simulink model "Controller"  (R2020b)
settings: Solver=FixedStepDiscrete  StartTime=0.0  StopTime=10.0  FixedStep=controllerSampleTime  RelTol=1e-3
values from neighbouring files (symbols this model uses):
  eetaRoad = 5.0    [AOTDataDictionary.sldd]
  egoAccMax = 5.0    [AOTDataDictionary.sldd]
  egoAccMin = -10.0    [AOTDataDictionary.sldd]
  egoSteerAngMax = 0.52359877559829882    [AOTDataDictionary.sldd]
  egoSteerAngMin = -0.52359877559829882    [AOTDataDictionary.sldd]
  egoVehLength = 4.948    [AOTDataDictionary.sldd]
  egoVehWidth = 2.009    [AOTDataDictionary.sldd]
  inflation_factor = 1.0    [AOTDataDictionary.sldd]
  L = 3.705    [AOTDataDictionary.sldd]
  l_F = 1.2525    [AOTDataDictionary.sldd]
  npcVehLength = 4.848    [AOTDataDictionary.sldd]
  npcVehWidth = 1.842    [AOTDataDictionary.sldd]
  obstcl_ellip_order = 6.0    [AOTDataDictionary.sldd]
  ReachableSetCurveResolution = 0.1    [AOTDataDictionary.sldd]
  RiskMaxValue = 100.0    [AOTDataDictionary.sldd]
  RiskValueThreshold = 15.0    [AOTDataDictionary.sldd]
  SenseResolution = 0.1    [AOTDataDictionary.sldd]
  v_des = 8.0    [AOTDataDictionary.sldd]
  XSenseRange = 20.0    [AOTDataDictionary.sldd]
  XSenseRangeArrSize = 401.0    [AOTDataDictionary.sldd]
  YSenseRange = 20.0    [AOTDataDictionary.sldd]
  YSenseRangeArrSize = 401.0    [AOTDataDictionary.sldd]
undefined symbols (not defined in the file or in its folder): VEH
libraries: mpclib x1, autolibshared x1, vehdynlibdriver x1
settings Model: DataDictionary=AOTDataDictionary.sldd  Creator=jiyoj  LastModifiedBy=jiyoj
settings DataIOCC: SaveOutput=off  SignalLogging=off  DSMLogging=off  SaveTime=off  ReturnWorkspaceOutputs=off

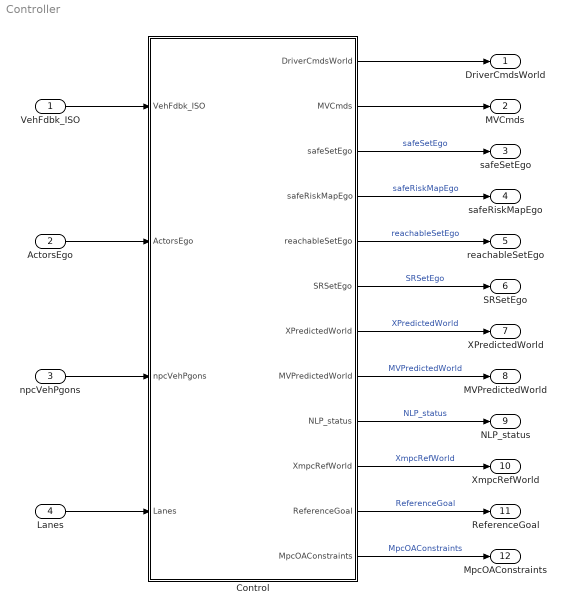
== system Controller ==
  VehFdbk_ISO : Inport  OutDataTypeStr=Bus: Veh_Fdbk  BusOutputAsStruct=on
  ActorsEgo : Inport  Port=2  OutDataTypeStr=Bus: BusActors  PortDimensions=[1 1]  BusOutputAsStruct=on
  npcVehPgons : Inport  Port=3  OutDataTypeStr=Bus: VehPgons  BusOutputAsStruct=on
  Lanes : Inport  Port=4  OutDataTypeStr=Bus: BusLaneBoundaries  PortDimensions=[1 1]  BusOutputAsStruct=on
  Control : Subsystem
  DriverCmdsWorld : Outport  OutDataTypeStr=Bus: DriverCmd  BusOutputAsStruct=on
  MVCmds : Outport  Port=2
  safeSetEgo : Outport  Port=3
  safeRiskMapEgo : Outport  Port=4
  reachableSetEgo : Outport  Port=5
  SRSetEgo : Outport  Port=6
  XPredictedWorld : Outport  Port=7
  MVPredictedWorld : Outport  Port=8
  NLP_status : Outport  Port=9
  XmpcRefWorld : Outport  Port=10
  ReferenceGoal : Outport  Port=11  OutDataTypeStr=Bus: Position2D  BusOutputAsStruct=on
  MpcOAConstraints : Outport  Port=12
  wires:
  VehFdbk_ISO/1 -> Control/1(VehFdbk_ISO)
  ActorsEgo/1 -> Control/2(ActorsEgo)
  Lanes/1 -> Control/4(Lanes)
  Control/1(DriverCmdsWorld) -> DriverCmdsWorld/1
  Control/3(safeSetEgo) -> safeSetEgo/1  "safeSetEgo"
  Control/4(safeRiskMapEgo) -> safeRiskMapEgo/1  "safeRiskMapEgo"
  npcVehPgons/1 -> Control/3(npcVehPgons)
  Control/5(reachableSetEgo) -> reachableSetEgo/1  "reachableSetEgo"
  Control/6(SRSetEgo) -> SRSetEgo/1  "SRSetEgo"
  Control/7(XPredictedWorld) -> XPredictedWorld/1  "XPredictedWorld"
  Control/8(MVPredictedWorld) -> MVPredictedWorld/1  "MVPredictedWorld"
  Control/9(NLP_status) -> NLP_status/1  "NLP_status"
  Control/10(XmpcRefWorld) -> XmpcRefWorld/1  "XmpcRefWorld"
  Control/11(ReferenceGoal) -> ReferenceGoal/1  "ReferenceGoal"
  Control/12(MpcOAConstraints) -> MpcOAConstraints/1  "MpcOAConstraints"
  Control/2(MVCmds) -> MVCmds/1

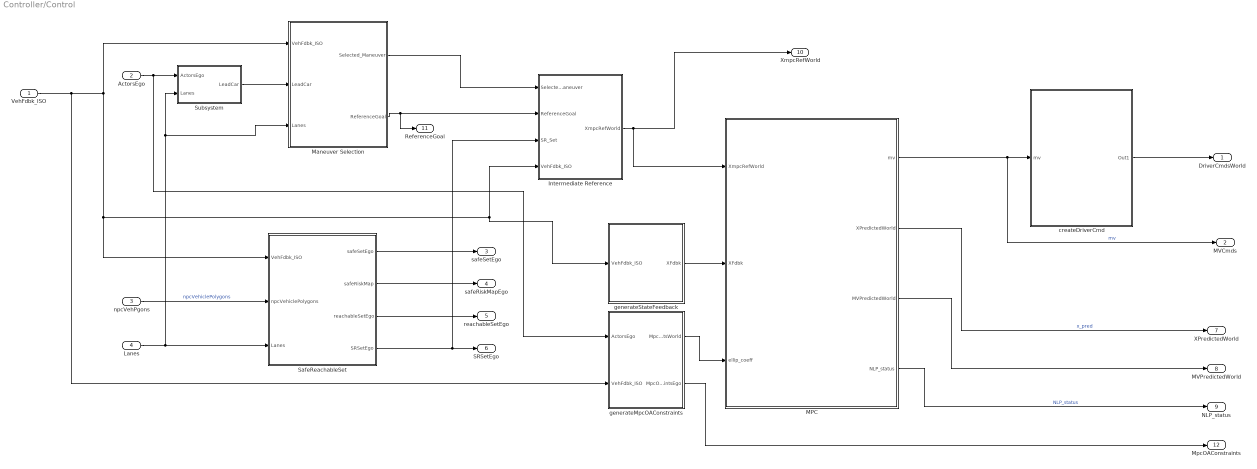
== system Controller/Control ==
  VehFdbk_ISO : Inport
  ActorsEgo : Inport  Port=2
  npcVehPgons : Inport  Port=3
  Lanes : Inport  Port=4
  Intermediate Reference : Subsystem
  MPC : Subsystem
  Maneuver Selection : Subsystem
  SafeReachableSet : Subsystem
  Subsystem : Subsystem
  createDriverCmd : Subsystem
  generateMpcOAConstraints : Subsystem
  generateStateFeedback : Subsystem
  DriverCmdsWorld : Outport
  MVCmds : Outport  Port=2
  safeSetEgo : Outport  Port=3
  safeRiskMapEgo : Outport  Port=4
  reachableSetEgo : Outport  Port=5
  SRSetEgo : Outport  Port=6
  XPredictedWorld : Outport  Port=7
  MVPredictedWorld : Outport  Port=8
  NLP_status : Outport  Port=9
  XmpcRefWorld : Outport  Port=10
  ReferenceGoal : Outport  Port=11
  MpcOAConstraints : Outport  Port=12
  wires:
  ActorsEgo/1 -> generateMpcOAConstraints/1(ActorsEgo), Subsystem/1(ActorsEgo)
  Lanes/1 -> SafeReachableSet/3(Lanes), Maneuver Selection/3(Lanes), Subsystem/2(Lanes)
  generateMpcOAConstraints/1(MpcOAConstraintsWorld) -> MPC/3(ellip_coeff)
  Maneuver Selection/1(Selected_Maneuver) -> Intermediate Reference/1(Selected_Maneuver)
  VehFdbk_ISO/1 -> generateMpcOAConstraints/2(VehFdbk_ISO), SafeReachableSet/1(VehFdbk_ISO), generateStateFeedback/1(VehFdbk_ISO), Intermediate Reference/4(VehFdbk_ISO), Maneuver Selection/1(VehFdbk_ISO)
  npcVehPgons/1 -> SafeReachableSet/2(npcVehiclePolygons)  "npcVehiclePolygons"
  SafeReachableSet/1(safeSetEgo) -> safeSetEgo/1
  SafeReachableSet/2(safeRiskMap) -> safeRiskMapEgo/1
  SafeReachableSet/3(reachableSetEgo) -> reachableSetEgo/1
  SafeReachableSet/4(SRSetEgo) -> SRSetEgo/1, Intermediate Reference/3(SR_Set)
  MPC/1(mv) -> MVCmds/1, createDriverCmd/1(mv)  "mv"
  createDriverCmd/1(Out1) -> DriverCmdsWorld/1
  Subsystem/1(LeadCar) -> Maneuver Selection/2(LeadCar)
  MPC/2(XPredictedWorld) -> XPredictedWorld/1  "x_pred"
  MPC/3(MVPredictedWorld) -> MVPredictedWorld/1
  MPC/4(NLP_status) -> NLP_status/1  "NLP_status"
  Maneuver Selection/2(ReferenceGoal) -> ReferenceGoal/1, Intermediate Reference/2(ReferenceGoal)
  generateMpcOAConstraints/2(MpcOAConstraintsEgo) -> MpcOAConstraints/1
  Intermediate Reference/1(XmpcRefWorld) -> MPC/1(XmpcRefWorld), XmpcRefWorld/1
  generateStateFeedback/1(XFdbk) -> MPC/2(XFdbk)

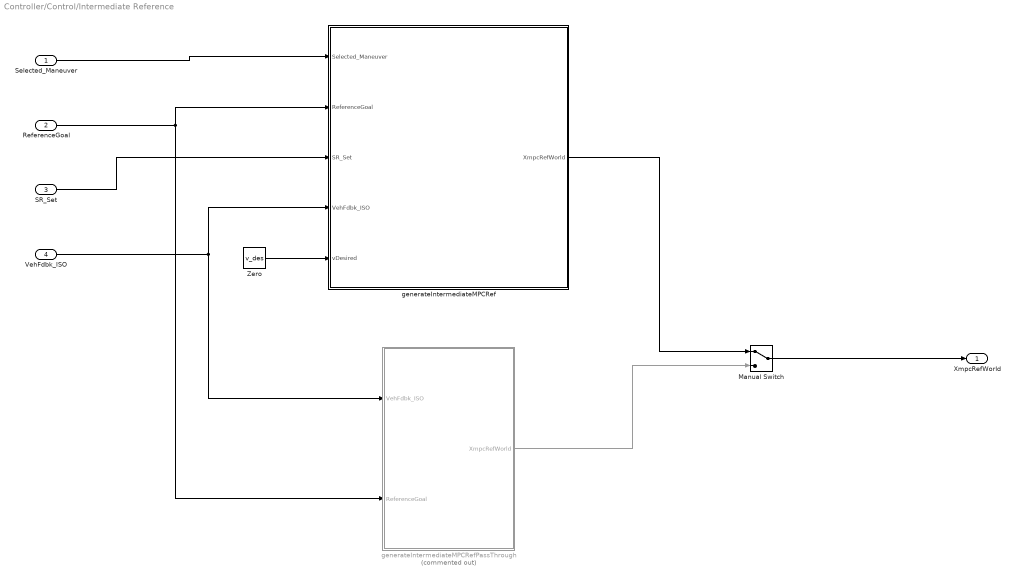
== system Controller/Control/Intermediate Reference ==
  Selected_Maneuver : Inport
  ReferenceGoal : Inport  Port=2
  SR_Set : Inport  Port=3
  VehFdbk_ISO : Inport  Port=4
  Manual Switch : ManualSwitch
  Zero : Constant  Value=v_des  OutDataTypeStr=Inherit: Inherit via back propagation
  generateIntermediateMPCRef : MATLAB Function  TreatAsAtomicUnit=on
  generateIntermediateMPCRefPassThrough : MATLAB Function  Commented=on  TreatAsAtomicUnit=on
  XmpcRefWorld : Outport
  wires:
  Selected_Maneuver/1 -> generateIntermediateMPCRef/1(Selected_Maneuver)
  SR_Set/1 -> generateIntermediateMPCRef/3(SR_Set)
  generateIntermediateMPCRef/1(XmpcRefWorld) -> Manual Switch/1
  ReferenceGoal/1 -> generateIntermediateMPCRefPassThrough/2(ReferenceGoal), generateIntermediateMPCRef/2(ReferenceGoal)
  generateIntermediateMPCRefPassThrough/1(XmpcRefWorld) -> Manual Switch/2
  VehFdbk_ISO/1 -> generateIntermediateMPCRefPassThrough/1(VehFdbk_ISO), generateIntermediateMPCRef/4(VehFdbk_ISO)
  Manual Switch/1 -> XmpcRefWorld/1
  Zero/1 -> generateIntermediateMPCRef/5(vDesired)

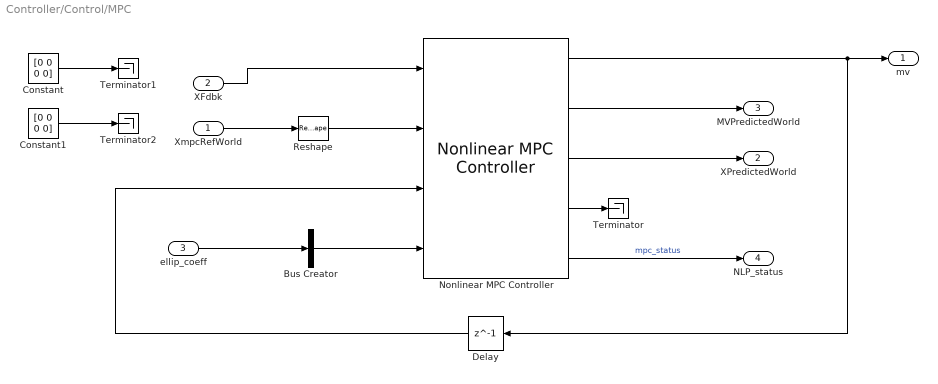
== system Controller/Control/MPC ==
  XmpcRefWorld : Inport
  XFdbk : Inport  Port=2
  ellip_coeff : Inport  Port=3
  Bus Creator : BusCreator  Inputs=1  OutDataTypeStr=Bus: MPCparams  NonVirtualBus=on
      settings: InheritFromInputs=off
  Constant : Constant  Value=[0 0 0 0]
  Constant1 : Constant  Value=[0 0 0 0]
  Delay : Delay  DelayLength=1
  Nonlinear MPC Controller : mpclib/Nonlinear MPC Controller  SCDEnableBlockLinearizationSpecification=on  nlmpcobj=mpc_planner  UseObjectTs=on  TsControl=-1  UseMEX=off  md_enabled=off  mvtarget_enabled=off  param_enabled=on  cost_enabled=off  mvseq_enabled=on  stateseq_enabled=on  ovseq_enabled=on  slack_enabled=off  status_enabled=on  ov_min=off  ov_max=off  mv_min=off  mv_max=off  mvrate_min=off  mvrate_max=off  state_min=off  state_max=off  ov_weight=off  mv_weight=off  mvrate_weight=off  ecr_weight=off  nlp_initialize=off
  Reshape : Reshape  OutputDimensionality=Row vector (2-D)
  Terminator : Terminator
  Terminator1 : Terminator
  Terminator2 : Terminator
  mv : Outport
  XPredictedWorld : Outport  Port=2
  MVPredictedWorld : Outport  Port=3
  NLP_status : Outport  Port=4
  wires:
  Nonlinear MPC Controller/5 -> NLP_status/1  "mpc_status"
  Nonlinear MPC Controller/2 -> MVPredictedWorld/1
  Nonlinear MPC Controller/3 -> XPredictedWorld/1
  ellip_coeff/1 -> Bus Creator/1
  Reshape/1 -> Nonlinear MPC Controller/2
  XmpcRefWorld/1 -> Reshape/1
  Bus Creator/1 -> Nonlinear MPC Controller/4
  Delay/1 -> Nonlinear MPC Controller/3
  XFdbk/1 -> Nonlinear MPC Controller/1
  Nonlinear MPC Controller/1 -> Delay/1, mv/1
  Nonlinear MPC Controller/4 -> Terminator/1
  Constant1/1 -> Terminator2/1
  Constant/1 -> Terminator1/1

== system Controller/Control/Maneuver Selection ==
  VehFdbk_ISO : Inport
  LeadCar : Inport  Port=2
  Lanes : Inport  Port=3
  Chart : Stateflow chart  TreatAsAtomicUnit=on
  Selected_Maneuver : Outport
  ReferenceGoal : Outport  Port=2
  wires:
  VehFdbk_ISO/1 -> Chart/1(VehFdbk_ISO)
  LeadCar/1 -> Chart/2(LeadCar)
  Chart/1(Selected_Maneuver) -> Selected_Maneuver/1
  Lanes/1 -> Chart/3(Lanes)
  Chart/2(ReferenceGoal) -> ReferenceGoal/1

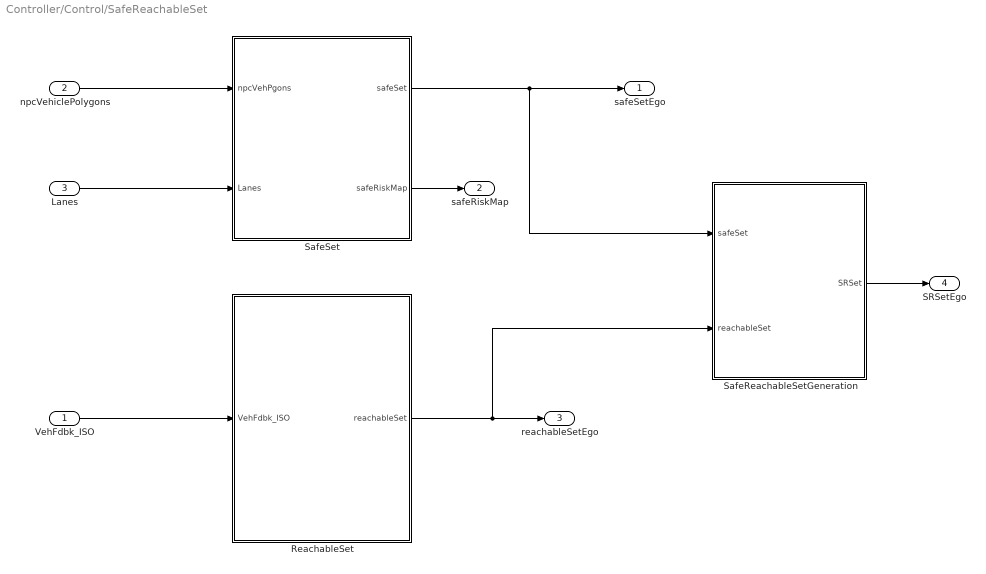
== system Controller/Control/SafeReachableSet ==
  VehFdbk_ISO : Inport
  npcVehiclePolygons : Inport  Port=2
  Lanes : Inport  Port=3
  ReachableSet : Subsystem
  SafeReachableSetGeneration : Subsystem
  SafeSet : Subsystem
  safeSetEgo : Outport
  safeRiskMap : Outport  Port=2
  reachableSetEgo : Outport  Port=3
  SRSetEgo : Outport  Port=4
  wires:
  npcVehiclePolygons/1 -> SafeSet/1(npcVehPgons)
  Lanes/1 -> SafeSet/2(Lanes)
  SafeSet/1(safeSet) -> SafeReachableSetGeneration/1(safeSet), safeSetEgo/1
  SafeSet/2(safeRiskMap) -> safeRiskMap/1
  VehFdbk_ISO/1 -> ReachableSet/1(VehFdbk_ISO)
  ReachableSet/1(reachableSet) -> SafeReachableSetGeneration/2(reachableSet), reachableSetEgo/1
  SafeReachableSetGeneration/1(SRSet) -> SRSetEgo/1

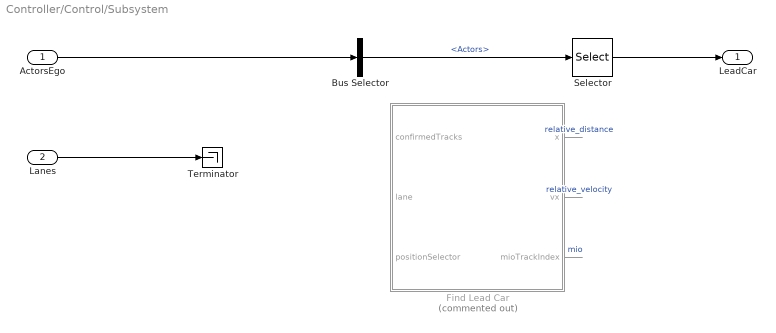
== system Controller/Control/Subsystem ==
  ActorsEgo : Inport
  Lanes : Inport  Port=2
  Bus Selector : BusSelector  OutputSignals=Actors
  Find Lead Car : MATLAB Function  Commented=on  TreatAsAtomicUnit=on
  Selector : Selector  InputPortWidth=2  IndexOptions=Index vector (dialog)  Indices=[1]  OutputSizes=1
  Terminator : Terminator
  LeadCar : Outport
  wires:
  ActorsEgo/1 -> Bus Selector/1
  Find Lead Car/2(vx) -> ?  "relative_velocity"
  Find Lead Car/3(mioTrackIndex) -> ?  "mio"
  Find Lead Car/1(x) -> ?  "relative_distance"
  Bus Selector/1 -> Selector/1  "<Actors>"
  Selector/1 -> LeadCar/1
  Lanes/1 -> Terminator/1

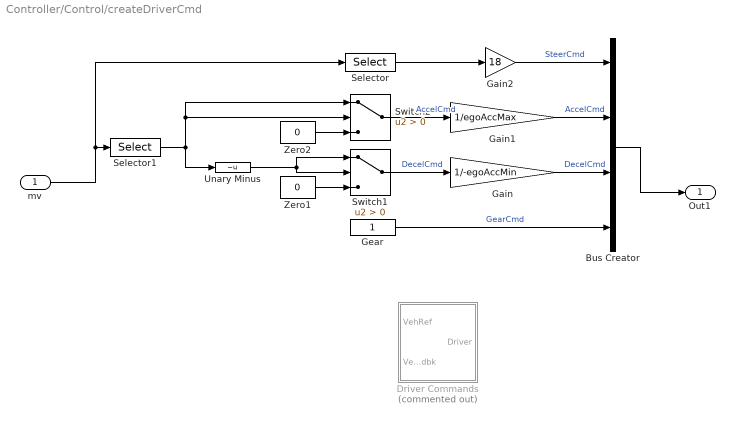
== system Controller/Control/createDriverCmd ==
  mv : Inport
  Bus Creator : BusCreator  Inputs=4  OutDataTypeStr=Bus: DriverCmd  NonVirtualBus=on
      settings: InheritFromInputs=off
  Driver Commands : Subsystem  Commented=on  VariantControl=0  mask{driverType=Longitudinal Driver}
      mask prompts: driverType "Vehicle command mode"
      mask init:
      | [~]=vdynblksdrvrconfig(gcb)
      settings: AttributesFormatString=%<driverType>
      mask Help: eval('vdynblkshelp(''vdcrdriver'')');
      mask TypeOptions driverType: Longitudinal Driver | Predictive Driver | Open Loop
      mask Display: image('driverlatlong.png');
  Gain : Gain  Gain=1/-egoAccMin
  Gain1 : Gain  Gain=1/egoAccMax
  Gain2 : Gain  Gain=18
  Gear : Constant
  Selector : Selector  InputPortWidth=2  IndexOptions=Index vector (dialog)  Indices=[2]  OutputSizes=1
  Selector1 : Selector  InputPortWidth=2  IndexOptions=Index vector (dialog)  Indices=[1]  OutputSizes=1
  Switch1 : Switch  Criteria=u2 > Threshold
  Switch2 : Switch  Criteria=u2 > Threshold
  Unary Minus : UnaryMinus
  Zero1 : Constant  Value=0  OutDataTypeStr=Inherit: Inherit via back propagation
  Zero2 : Constant  Value=0  OutDataTypeStr=Inherit: Inherit via back propagation
  Out1 : Outport
  wires:
  mv/1 -> Selector/1, Selector1/1
  Bus Creator/1 -> Out1/1
  Gear/1 -> Bus Creator/4  "GearCmd"
  Selector/1 -> Gain2/1
  Switch2/1 -> Gain1/1  "AccelCmd"
  Zero1/1 -> Switch1/3
  Switch1/1 -> Gain/1  "DecelCmd"
  Selector1/1 -> Switch2/1, Switch2/2, Unary Minus/1
  Zero2/1 -> Switch2/3
  Unary Minus/1 -> Switch1/2, Switch1/1
  Gain/1 -> Bus Creator/3  "DecelCmd"
  Gain1/1 -> Bus Creator/2  "AccelCmd"
  Gain2/1 -> Bus Creator/1  "SteerCmd"

== system Controller/Control/generateMpcOAConstraints ==
  ActorsEgo : Inport
  VehFdbk_ISO : Inport  Port=2
  Manual Switch : ManualSwitch
  Zero : Constant  Value=[0 0 0 0 0 obstcl_ellip_order ]  VectorParams1D=off  OutDataTypeStr=Inherit: Inherit via back propagation
  generateMpcOAConstraintsProxy : MATLAB Function  TreatAsAtomicUnit=on
  MpcOAConstraintsWorld : Outport
  MpcOAConstraintsEgo : Outport  Port=2
  wires:
  Zero/1 -> Manual Switch/2
  Manual Switch/1 -> MpcOAConstraintsWorld/1
  generateMpcOAConstraintsProxy/1(MpcOAConstraintsWorld) -> Manual Switch/1
  VehFdbk_ISO/1 -> generateMpcOAConstraintsProxy/2(VehFdbk_ISO)
  ActorsEgo/1 -> generateMpcOAConstraintsProxy/1(ActorsEgo)
  generateMpcOAConstraintsProxy/2(MpcOAConstraintsEgo) -> MpcOAConstraintsEgo/1

== system Controller/Control/generateStateFeedback ==
  VehFdbk_ISO : Inport
  Bus Selector : BusSelector  OutputSignals=Position.X,Position.Y,Orientation.psi
  Bus Selector1 : BusSelector  OutputSignals=Velocity.Xdot,Velocity.Ydot
  Vector Concatenate : Concatenate  NumInputs=4
  Velocity : Subsystem
  XFdbk : Outport
  wires:
  VehFdbk_ISO/1 -> Bus Selector1/1, Bus Selector/1
  Bus Selector1/1 -> Velocity/1(Vx)  "<Xdot>"
  Bus Selector1/2 -> Velocity/2(Vy)  "<Ydot>"
  Velocity/1(v) -> Vector Concatenate/4
  Bus Selector/1 -> Vector Concatenate/1  "<X>"
  Bus Selector/2 -> Vector Concatenate/2  "<Y>"
  Bus Selector/3 -> Vector Concatenate/3  "<psi>"
  Vector Concatenate/1 -> XFdbk/1  "x_curr"

== system Controller/Control/SafeReachableSet/ReachableSet ==
  VehFdbk_ISO : Inport
  generateReachableSetProxy : MATLAB Function  TreatAsAtomicUnit=on
  reachableSet : Outport
  wires:
  VehFdbk_ISO/1 -> generateReachableSetProxy/1(VehFdbk_ISO)
  generateReachableSetProxy/1(reachableSet) -> reachableSet/1

== system Controller/Control/SafeReachableSet/SafeReachableSetGeneration ==
  safeSet : Inport
  reachableSet : Inport  Port=2
  getSRSetProxy : MATLAB Function  TreatAsAtomicUnit=on
  SRSet : Outport
  wires:
  safeSet/1 -> getSRSetProxy/1(safeSet)
  reachableSet/1 -> getSRSetProxy/2(reachableSet)
  getSRSetProxy/1(SRSet) -> SRSet/1

== system Controller/Control/SafeReachableSet/SafeSet ==
  npcVehPgons : Inport
  Bus Element In : Inport  Port=2  PortName=Lanes  Element=LaneBoundaries
  generateSafeSetProxy : MATLAB Function  TreatAsAtomicUnit=on
  safeSet : Outport
  safeRiskMap : Outport  Port=2
  wires:
  npcVehPgons/1 -> generateSafeSetProxy/1(npcVehPgons)
  generateSafeSetProxy/2(safeRiskMap) -> safeRiskMap/1
  generateSafeSetProxy/1(safeSet) -> safeSet/1
  Bus Element In/1 -> generateSafeSetProxy/2(Lane)

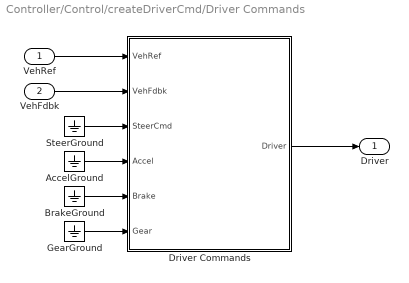
== system Controller/Control/createDriverCmd/Driver Commands ==
  VehRef : Inport
  VehFdbk : Inport  Port=2
  AccelGround : Ground
  BrakeGround : Ground
  Driver Commands : Subsystem  Variant=on  VariantControlMode=label  VariantControl=Variant1  LabelModeActiveChoice=0  AllowZeroVariantControls=on
  GearGround : Ground
  SteerGround : Ground
  Driver : Outport  VectorParamsAs1DForOutWhenUnconnected=off
  wires:
  VehRef/1 -> Driver Commands/1(VehRef)
  VehFdbk/1 -> Driver Commands/2(VehFdbk)
  Driver Commands/1(" Driver") -> Driver/1
  SteerGround/1 -> Driver Commands/3(SteerCmd)
  AccelGround/1 -> Driver Commands/4(Accel)
  BrakeGround/1 -> Driver Commands/5(Brake)
  GearGround/1 -> Driver Commands/6(Gear)

== system Controller/Control/generateStateFeedback/Velocity ==
  Vx : Inport
  Vy : Inport  Port=2
  Add : Sum
  Sqrt : Sqrt  SaturateOnIntegerOverflow=on
  Square : Math  Operator=square  SaturateOnIntegerOverflow=on
  Square1 : Math  Operator=square  SaturateOnIntegerOverflow=on
  v : Outport
  wires:
  Vy/1 -> Square1/1
  Vx/1 -> Square/1
  Sqrt/1 -> v/1
  Square1/1 -> Add/2
  Add/1 -> Sqrt/1
  Square/1 -> Add/1

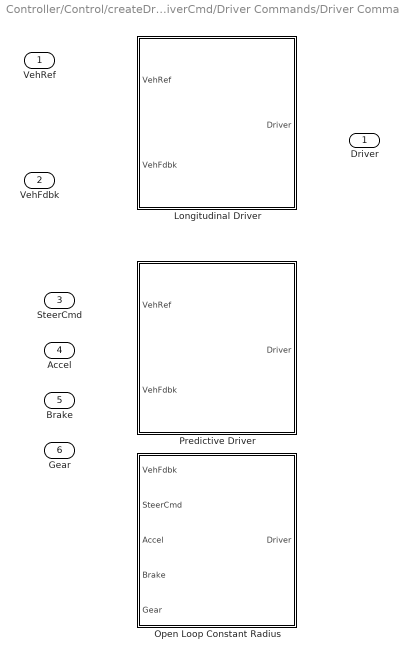
== system Controller/Control/createDriverCmd/Driver Commands/Driver Commands ==
  VehRef : Inport
  VehFdbk : Inport  Port=2
  SteerCmd : Inport  Port=3
  Accel : Inport  Port=4
  Brake : Inport  Port=5
  Gear : Inport  Port=6
  Longitudinal Driver : Subsystem  VariantControl=0
  Open Loop Constant Radius : Subsystem  VariantControl=2
  Predictive Driver : Subsystem  VariantControl=1
  " Driver" : Outport  VectorParamsAs1DForOutWhenUnconnected=off

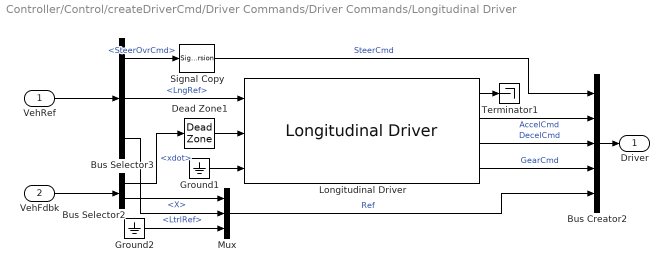
== system Controller/Control/createDriverCmd/Driver Commands/Driver Commands/Longitudinal Driver ==
  VehRef : Inport
  VehFdbk : Inport  Port=2
  Bus Creator2 : BusCreator  Inputs=5
  Bus Selector2 : BusSelector  OutputSignals=Body.BdyFrm.Cg.Vel.xdot,Body.InertFrm.Cg.Disp.X
  Bus Selector3 : BusSelector  OutputSignals=SteerOvrCmd,LngRef,LtrlRef
  Dead Zone1 : DeadZone  LowerValue=-.1  UpperValue=.1  SaturateOnIntegerOverflow=on
  Ground1 : Ground
  Ground2 : Ground
  Longitudinal Driver : autolibshared/Longitudinal Driver  extAccelOvr=off  extDecelOvr=off  extAccelHld=off  extDecelHld=off  extAccelZero=off  extDecelZero=off  cntrlType=Predictive  shftType=Reverse, Neutral, Drive  velUnits=m/s  gearOut=on  Kp=5  Ki=5  Kff=.1  Kg=0  VehVelVec=[0 100]  KffVec=[.1 .1]  KpVec=[10 10]  KiVec=[5 5]  KgVec=[0 0]  m=VEH.Mass  Kpt=3000  tau=.5  L=2  aR=200  bR=2.5  cR=.5  g=9.81  vnom=5  Kaw=1  tauerr=.1  tauPt=2  GearInit=0  tShift=.1  pdlVec=[0.1 0.4 0.5 0.9]  upShftTbl=[-1 12.9375 26.4375 39.9375 51.18749999999999 62.4375 72.84375 83.25;-1 16.3125 29.8125 43.3125 54.5624 65.8125 76.78125 87.75;-1 19.6875 33.1875 46.68749999999999 57.9375 69.1875 80.71875 92.25;-1 33 52.5 77.25 100.5 138.75 161.875 185]  dwnShftTbl=[1 9.5625 23.0625 36.5625 47.8125 59.0625 68.90625 78.75;1 12.9375 26.4375 39.9375 51.18749999999999 62.4375 72.84375 83.25;1 16.3125 29.8125 43.3125 54.562499 65.8125 76.78125 87.75;1 19.6875 33.1875 46.68749999999999 57.9375 69.1875 80.71875 92.25]  tClutch=.5  tRev=.5  tPark=120  aMode=2  UpGearVec="[0  1  2  3  4  5  6  7]"  DownGearVec="[1  2  3  4  5  6  7  8]"
      settings: SourceProductBaseCode=PW,MT,UV,VE,VP
  Mux : Mux  Inputs=3
  Signal Copy : SignalConversion  OverrideOpt=off
  Terminator1 : Terminator
  Driver : Outport  VectorParamsAs1DForOutWhenUnconnected=off
  wires:
  VehRef/1 -> Bus Selector3/1
  Signal Copy/1 -> Bus Creator2/1  "SteerCmd"
  Longitudinal Driver/2 -> Bus Creator2/2  "AccelCmd"
  Dead Zone1/1 -> Longitudinal Driver/2
  Bus Selector3/2 -> Longitudinal Driver/1  "<LngRef>"
  Ground1/1 -> Longitudinal Driver/3
  Bus Selector2/1 -> Dead Zone1/1  "<xdot>"
  Bus Creator2/1 -> Driver/1
  Longitudinal Driver/1 -> Terminator1/1
  Longitudinal Driver/3 -> Bus Creator2/3  "DecelCmd"
  VehFdbk/1 -> Bus Selector2/1
  Bus Selector3/1 -> Signal Copy/1  "<SteerOvrCmd>"
  Ground2/1 -> Mux/3
  Bus Selector2/2 -> Mux/1  "<X>"
  Mux/1 -> Bus Creator2/5  "Ref"
  Bus Selector3/3 -> Mux/2  "<LtrlRef>"
  Longitudinal Driver/4 -> Bus Creator2/4  "GearCmd"

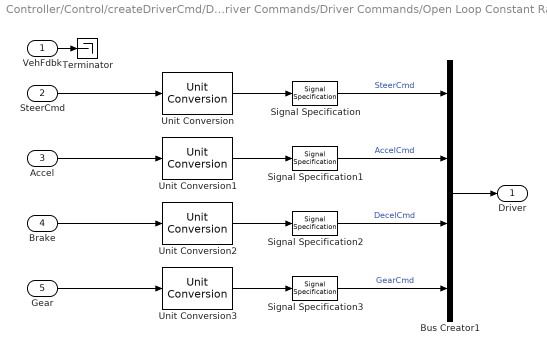
== system Controller/Control/createDriverCmd/Driver Commands/Driver Commands/Open Loop Constant Radius ==
  VehFdbk : Inport
  SteerCmd : Inport  Port=2
  Accel : Inport  Port=3  Unit=one
  Brake : Inport  Port=4  Unit=1
  Gear : Inport  Port=5  Unit=1
  Bus Creator1 : BusCreator  Inputs=4
  Signal Specification : SignalSpecification  Unit=rad
  Signal Specification1 : SignalSpecification  Unit=1
  Signal Specification2 : SignalSpecification  Unit=1
  Signal Specification3 : SignalSpecification  Unit=1
  Terminator : Terminator
  Unit Conversion{,1..3} (4 alike) : UnitConversion
  Driver : Outport  VectorParamsAs1DForOutWhenUnconnected=off
  wires:
  Unit Conversion3/1 -> Signal Specification3/1
  Unit Conversion2/1 -> Signal Specification2/1
  Unit Conversion/1 -> Signal Specification/1
  Bus Creator1/1 -> Driver/1
  Accel/1 -> Unit Conversion1/1
  VehFdbk/1 -> Terminator/1
  SteerCmd/1 -> Unit Conversion/1
  Unit Conversion1/1 -> Signal Specification1/1
  Brake/1 -> Unit Conversion2/1
  Gear/1 -> Unit Conversion3/1
  Signal Specification/1 -> Bus Creator1/1  "SteerCmd"
  Signal Specification1/1 -> Bus Creator1/2  "AccelCmd"
  Signal Specification2/1 -> Bus Creator1/3  "DecelCmd"
  Signal Specification3/1 -> Bus Creator1/4  "GearCmd"

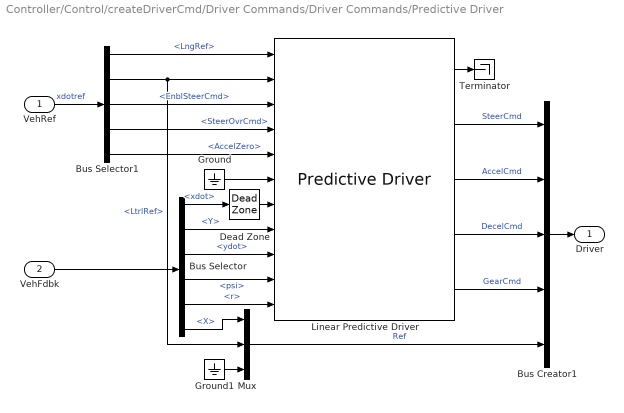
== system Controller/Control/createDriverCmd/Driver Commands/Driver Commands/Predictive Driver ==
  VehRef : Inport
  VehFdbk : Inport  Port=2
  Bus Creator1 : BusCreator  Inputs=5
  Bus Selector : BusSelector  OutputSignals=Body.BdyFrm.Cg.Vel.xdot,Body.InertFrm.Cg.Disp.Y,Body.BdyFrm.Cg.Vel.ydot,Body.InertFrm.Cg.Ang.psi,Body.BdyFrm.Cg.AngVel.r,Body.InertFrm.Cg.Disp.X
  Bus Selector1 : BusSelector  OutputSignals=LngRef,LtrlRef,EnblSteerCmd,SteerOvrCmd,AccelZero
  Dead Zone : DeadZone  LowerValue=-.5  UpperValue=.5  ZeroCross=off  SaturateOnIntegerOverflow=on
  Ground : Ground
  Ground1 : Ground
  Linear Predictive Driver : vehdynlibdriver/Predictive Driver  extAccelOvr=off  extDecelOvr=off  extAccelHld=off  extDecelHld=off  extAccelZero=on  extDecelZero=off  extSteerOvr=on  extSteerHld=off  extSteerZero=off  cntrlType=Predictive  cntrlTypeLat=Predictive  shftType=Reverse, Neutral, Drive  coordMode=SAE J670 (Z-down)  velUnits=m/s  angUnits=rad  gearOut=on  steerOut=on  Kp=3  Ki=1  Kff=1  Kg=0  VehVelVec=[0 100]  KffVec=[.1 .1]  KpVec=[10 10]  KiVec=[5 5]  KgVec=[0 0]  vnom=5  Kaw=1  tauerr=.075  tau=.15  L=6  Kpt=15000  aR=200  bR=2.5  cR=.5  g=9.81  vecPose=off  dynamMode=on  PositionGainF=2.5  PositionGainR=2.5  YawRateGain=.2  DelayGain=.2  a=VEH.FrontAxlePositionfromCG  b=VEH.RearAxlePositionfromCG  m=VEH.Mass  Cy_f=5000  Cy_r=7000  I=VEH.YawMomentInertia  Ksteer=18  theta=40*pi/180  GearInit=0  tShift=.1  pdlVec=[0.1 0.4 0.5 0.9]  upShftTbl=[-1 12.9375 26.4375 39.9375 51.18749999999999 62.4375 72.84375 83.25;-1 16.3125 29.8125 43.3125 54.5624 65.8125 76.78125 87.75;-1 19.6875 33.1875 46.68749999999999 57.9375 69.1875 80.71875 92.25;-1 33 52.5 77.25 100.5 138.75 161.875 185]  dwnShftTbl=[-1 12.9375 26.4375 39.9375 51.18749999999999 62.4375 72.84375 83.25;-1 16.3125 29.8125 43.3125 54.5624 65.8125 76.78125 87.75;-1 19.6875 33.1875 46.68749999999999 57.9375 69.1875 80.71875 92.25;-1 33 52.5 77.25 100.5 138.75 161.875 185]  tClutch=.5  tRev=.5  tPark=120  UpGearVec="[0  1  2  3  4  5  6  7]"  DownGearVec="[1  2  3  4  5  6  7  8]"  aMode=2
      settings: SourceProductBaseCode=VE
  Mux : Mux  Inputs=3
  Terminator : Terminator
  Driver : Outport  VectorParamsAs1DForOutWhenUnconnected=off
  wires:
  Mux/1 -> Bus Creator1/5  "Ref"
  Bus Selector/6 -> Mux/1  "<X>"
  Linear Predictive Driver/5 -> Bus Creator1/4  "GearCmd"
  Bus Selector/3 -> Linear Predictive Driver/9  "<ydot>"
  Linear Predictive Driver/1 -> Terminator/1
  Bus Selector/5 -> Linear Predictive Driver/11  "<r>"
  Bus Selector1/2 -> Mux/2, Linear Predictive Driver/2  "<LtrlRef>"
  Ground1/1 -> Mux/3
  Ground/1 -> Linear Predictive Driver/6
  Bus Selector/1 -> Dead Zone/1  "<xdot>"
  Bus Selector/4 -> Linear Predictive Driver/10  "<psi>"
  Linear Predictive Driver/4 -> Bus Creator1/3  "DecelCmd"
  Dead Zone/1 -> Linear Predictive Driver/7
  VehFdbk/1 -> Bus Selector/1
  VehRef/1 -> Bus Selector1/1  "xdotref"
  Linear Predictive Driver/2 -> Bus Creator1/1  "SteerCmd"
  Bus Creator1/1 -> Driver/1
  Linear Predictive Driver/3 -> Bus Creator1/2  "AccelCmd"
  Bus Selector/2 -> Linear Predictive Driver/8  "<Y>"
  Bus Selector1/1 -> Linear Predictive Driver/1  "<LngRef>"
  Bus Selector1/5 -> Linear Predictive Driver/5  "<AccelZero>"
  Bus Selector1/3 -> Linear Predictive Driver/3  "<EnblSteerCmd>"
  Bus Selector1/4 -> Linear Predictive Driver/4  "<SteerOvrCmd>"

== matlab function Controller/Control/SafeReachableSet/ReachableSet/generateReachableSetProxy ==
  data: tf parameter; egoAccMin parameter; egoAccMax parameter; egoSteerAngMin parameter; egoSteerAngMax parameter; v_des parameter; L parameter; l_F parameter; ReachableSetCurveResolution parameter; VehFdbk_ISO input; reachableSet output size=[ReachableSet_MaxVertices 2]
function reachableSet = fcn(tf, egoAccMin, egoAccMax, egoSteerAngMin, egoSteerAngMax, v_des, L, l_F, ReachableSetCurveResolution,...
                            VehFdbk_ISO)
reachableSet = zeros(200, 2);
XFdbk = [VehFdbk_ISO.Position.X, VehFdbk_ISO.Position.Y, VehFdbk_ISO.Orientation.psi, VehFdbk_ISO.Velocity.Xdot];
coder.extrinsic('generateReachableSet')
reachableSet = generateReachableSet(tf, egoAccMin, egoAccMax, egoSteerAngMin, egoSteerAngMax, v_des, L, l_F,ReachableSetCurveResolution, XFdbk);

== matlab function Controller/Control/SafeReachableSet/SafeReachableSetGeneration/getSRSetProxy ==
  data: safeSet input; reachableSet input; SRSet output size=[XSenseRangeArrSize*YSenseRangeArrSize 2]; YSenseRangeArrSize parameter; XSenseRangeArrSize parameter
function SRSet = fcn(safeSet, reachableSet, YSenseRangeArrSize, XSenseRangeArrSize)
SRSet = zeros(XSenseRangeArrSize*YSenseRangeArrSize,2);
SRSet = generateSRSet(safeSet,reachableSet);

== matlab function Controller/Control/Intermediate Reference/generateIntermediateMPCRef ==
  data: Selected_Maneuver input; ReferenceGoal input; SR_Set input; XmpcRefWorld output; VehFdbk_ISO input; vDesired input
function XmpcRefWorld = fcn(Selected_Maneuver, ReferenceGoal, SR_Set, VehFdbk_ISO, vDesired)


[~, maxDistLocationIndex]  = min(vecnorm(bsxfun(@minus, SR_Set,[ReferenceGoal.X, ReferenceGoal.Y]),2,2));

inputPose.X = SR_Set(maxDistLocationIndex,1); inputPose.Y = SR_Set(maxDistLocationIndex,2); inputPose.Z = 0;
%Transform to World for MPC Trajectory Planning 
outputPose = transformEgo(inputPose, VehFdbk_ISO.Position, VehFdbk_ISO.Orientation, 1);
XmpcRefWorld = [outputPose.X outputPose.Y 0 vDesired];

== matlab function Controller/Control/Intermediate Reference/generateIntermediateMPCRefPassThrough ==
  data: XmpcRefWorld output size=[1 4]; VehFdbk_ISO input; ReferenceGoal input
function XmpcRefWorld = fcn(VehFdbk_ISO, ReferenceGoal)

inputPose.X = ReferenceGoal.X; inputPose.Y =  ReferenceGoal.Y; inputPose.Z = 0;

%Transform to World for MPC Trajectory Planning 
outputPose = transformEgo(inputPose, VehFdbk_ISO.Position, VehFdbk_ISO.Orientation, 1);
XmpcRefWorld = [outputPose.X outputPose.Y 0 15];

== matlab function Controller/Control/generateMpcOAConstraints/generateMpcOAConstraintsProxy ==
  data: npcVehLength parameter; npcVehWidth parameter; egoVehLength parameter; egoVehWidth parameter; obstcl_ellip_order parameter; inflation_factor parameter; ActorsEgo input; MpcOAConstraintsWorld output; VehFdbk_ISO input; MpcOAConstraintsEgo output
function [MpcOAConstraintsWorld, MpcOAConstraintsEgo]   = fcn(npcVehLength, npcVehWidth,egoVehLength, egoVehWidth, obstcl_ellip_order,inflation_factor,...
    ActorsEgo, VehFdbk_ISO)

MpcOAConstraintsWorld = [0 0 0 0 0 1];
MpcOAConstraintsEgo = MpcOAConstraintsWorld;

npcVeh1Ego.Position = ActorsEgo.Actors(1).Position;
npcVeh1Ego.Orientation = deg2rad([ActorsEgo.Actors(1).Roll ActorsEgo.Actors(1).Pitch ActorsEgo.Actors(1).Yaw]);
% Generate ellipse coefficients in Ego Frame
f = nthroot(2,obstcl_ellip_order);
MpcOAConstraintsEgo(1:5) = [ f*((egoVehLength + npcVehLength)/2)*inflation_factor,...
    f*((egoVehWidth + npcVehWidth)/2)*inflation_factor,...
    npcVeh1Ego.Position(1,1), npcVeh1Ego.Position(1,2), -npcVeh1Ego.Orientation(1,3)];
MpcOAConstraintsEgo(6) = obstcl_ellip_order;

% Generate ellipse coefficients in World Frame
egoVeh.Position = [VehFdbk_ISO.Position.X VehFdbk_ISO.Position.Y VehFdbk_ISO.Position.Z];
egoVeh.Orientation = [VehFdbk_ISO.Orientation.phi VehFdbk_ISO.Orientation.theta VehFdbk_ISO.Orientation.psi];
rotMatE2N = eul2rotm(npcVeh1Ego.Orientation, 'XYZ');
rotMatW2E = eul2rotm(egoVeh.Orientation, 'XYZ');
transformMatE2N = [[rotMatE2N;0 0 0], [npcVeh1Ego.Position 1]'];
transformMatW2E = [[rotMatW2E;0 0 0], [egoVeh.Position 1]'];
transformN2W = transformMatW2E*transformMatE2N;
npcVeh1World.Position = transformN2W(1:3, 4)';
npcVeh1World.Orientation = rotm2eul(transformN2W(1:3, 1:3), 'XYZ');

% Generate ellipse coefficients
f = nthroot(2,obstcl_ellip_order);
MpcOAConstraintsWorld(1:5) = [ f*((egoVehLength + npcVehLength)/2)*inflation_factor,...
    f*((egoVehWidth + npcVehWidth)/2)*inflation_factor,...
    npcVeh1World.Position(1,1), npcVeh1World.Position(1,2), -npcVeh1World.Orientation(1,3)];
MpcOAConstraintsWorld(6) = obstcl_ellip_order;

== matlab function Controller/Control/SafeReachableSet/SafeSet/generateSafeSetProxy ==
  data: safeSet output size=[XSenseRangeArrSize*YSenseRangeArrSize 2]; npcVehPgons input Bus: VehPgons; Lane input Bus: BusLaneBoundariesLaneBoundaries; safeRiskMap output size=[XSenseRangeArrSize YSenseRangeArrSize]; YSenseRangeArrSize parameter; XSenseRangeArrSize parameter; YSenseRange parameter; XSenseRange parameter; SenseResolution parameter; RiskMaxValue parameter; RiskValueThreshold parameter; eetaRoad parameter
function [safeSet, safeRiskMap] = fcn(npcVehPgons, Lane, YSenseRangeArrSize, XSenseRangeArrSize, YSenseRange, XSenseRange, SenseResolution, RiskMaxValue,  RiskValueThreshold, eetaRoad)
safeRiskMap = zeros(XSenseRangeArrSize,YSenseRangeArrSize);
safeSet = zeros(XSenseRangeArrSize*YSenseRangeArrSize, 2);
coder.extrinsic('generateSafeSet')
[safeSet, safeRiskMap] = generateSafeSet(npcVehPgons,Lane, XSenseRange, YSenseRange, SenseResolution, XSenseRangeArrSize, YSenseRangeArrSize, RiskMaxValue, RiskValueThreshold, eetaRoad);

== matlab function Controller/Control/Subsystem/Find Lead Car ==
  data: confirmedTracks input; x output size=[1 1]; vx output size=[1 1]; lane input; mioTrackIndex output; positionSelector input
function [x,vx,mioTrackIndex] = findLeadCar(confirmedTracks, lane, positionSelector)
% This function finds the lead car: a car in front of the ego car that
% satisfies all the criteria below:
% * Within the ego car's lane.
% * In front of the ego car.
% * Closest to the ego car.

% Note: If you change state definition, change the following:
%       State = [x;vx;y;vy;z;vz] (3D constant velocity)
numStates = 6;

% Initialize outputs and parameters
maxX = cast(1000, 'like', confirmedTracks.Tracks(1).State);  % Far enough forward so that no track is expected to exceed this distance
mioTrackIndex = 0;

% If lane detection is not available, the ego car is assumed to be located
% in the middle of its lane. The lane width is assumed to be 3.6m, typical
% highway lane width.
laneWidth = 3.6;
halfLaneWidth = laneWidth/2;

if lane.Left.Strength > 0.01
    lb = [lane.Left.CurvatureDerivative/6,...
        lane.Left.Curvature/2,...
        lane.Left.HeadingAngle,...
        lane.Left.LateralOffset];
else
    lb = single([0,0,0,halfLaneWidth]);
end

if lane.Right.Strength > 0.01
    rb = [lane.Right.CurvatureDerivative/6,...
        lane.Right.Curvature/2,...
        lane.Right.HeadingAngle,...
        lane.Right.LateralOffset];
else
    rb = single([0,0,0,-halfLaneWidth]);    
end

for i = 1:confirmedTracks.NumTracks
    position = positionSelector * confirmedTracks.Tracks(i).State;
    x = position(1); % Longitudinal position of the track relative to ego
    y = position(2); % Lateral position of the track relative to ego
    
    if x < maxX && x > 0 % No point checking otherwise

        yleftLane  = polyval(lb,x); % lateral position of left lane
        yrightLane = polyval(rb,x); % lateral position of right lane
        
        % Find a new lead car
        if (yrightLane <= y) && (y <= yleftLane)
            maxX = x;
            mioTrackIndex(:) = i;
        end
    end
end

if mioTrackIndex>0
    mioState = confirmedTracks.Tracks(mioTrackIndex).State;
else
    mioState = inf(numStates,1,'like',confirmedTracks.Tracks(1).State);
end

% Output:
x = mioState(1);    % Longitudinal position of the lead car
vx = mioState(2);   % Longitudinal velocity of the lead car

== stateflow chart Controller/Control/Maneuver Selection/Chart ==
  state Overtaking
    Selected_Maneuver = CurrentManeuver.Overtake
    state Overtaking
      ReferenceGoal.X = LeadCar.Position(1,1) + d_overtake
      [ReferenceGoal.Y, LaneIndexY] = getfinalRefY(Lanes,ReferenceGoal.X );
      ReferenceGoal.X = Lanes.LaneBoundaries(6).Coordinates(LaneIndexY,1);
    state OvertakeComplete
    (default) -> Overtaking.Overtaking
    Overtaking.Overtaking -> OvertakeComplete : [checkOvertakeSuccess(VehFdbk_ISO,LeadCar)]
  state LaneKeeping
    Selected_Maneuver = CurrentManeuver.LaneKeep;
    ReferenceGoal.X = d_lanekeep;
    [ReferenceGoal.Y, LaneIndexY] = getfinalRefY(Lanes,ReferenceGoal.X );
    ReferenceGoal.X = Lanes.LaneBoundaries(6).Coordinates(LaneIndexY,1);
  state AbortOvertaking [commented out]
    ReferenceGoal.X = LeadCar.Position(1,1) - d_overtake
    [ReferenceGoal.Y, LaneIndexY] = getfinalRefY(Lanes,ReferenceGoal.X );
    ReferenceGoal.X = Lanes.LaneBoundaries(6).Coordinates(LaneIndexY,1);
  (default) -> LaneKeeping
  LaneKeeping -> Overtaking : [LeadCar.Position(1,1) < d_overtake &&...
      |  LeadCar.Position(1,1) > 0]
  OvertakeComplete -> LaneKeeping
  Overtaking -> (junction 51) [commented out] : after(1,sec)
  (junction 51) -> AbortOvertaking [commented out]
  data: VehFdbk function_input; overtakeComplete function_output; OvertakenLeadCar function_input; LanesInfo function_input; finalRefY function_output; X function_input; LaneIndex function_output; Selected_Maneuver output Enum: CurrentManeuver; VehFdbk_ISO input; LeadCar input; d_overtake constant double =15; Lanes input; d_lanekeep constant double =10; ReferenceGoal output Bus: Position2D; LaneIndexY local
  function overtakeComplete = checkOvertakeSuccess(VehFdbk, OvertakenLeadCar):
    | function overtakeComplete = checkOvertakeSuccess(VehFdbk, OvertakenLeadCar)
    | 
    | if OvertakenLeadCar.Position(1,1) < 0 &&...
    |         Lanes.LaneBoundaries(6).LateralOffset < 0 &&...
    |         Lanes.LaneBoundaries(5).LateralOffset > 0
    |     
    |     overtakeComplete = true;
    | else
    |     overtakeComplete = false;
    | end
  function [finalRefY, LaneIndex] = getfinalRefY(LanesInfo,X):
    | function [finalRefY, LaneIndex] = getfinalRefY(LanesInfo,X)
    | LaneXCoordinates = LanesInfo.LaneBoundaries(6).Coordinates(:,1);
    | LaneIndex = find(abs(LaneXCoordinates-X) < 0.1);
    | if isempty(LaneIndex)
    |     LaneIndex = length(LaneXCoordinates);
    | else
    |     LaneIndex = LaneIndex(1);
    | end
    | finalRefY = LanesInfo.LaneBoundaries(6).Coordinates(LaneIndex,2) - ((LanesInfo.LaneBoundaries(6).Coordinates(LaneIndex,2)-LanesInfo.LaneBoundaries(5).Coordinates(LaneIndex,2))/2);  
    | % finalRefY = 0;
    | end
